simulink model "exp11_4"  (R2020a)
settings: Solver=FixedStepAuto  StartTime=0.0  StopTime=5  FixedStep=0.01  RelTol=1e-3
settings Model: Creator=Sing Ngai  LastModifiedBy=zengw

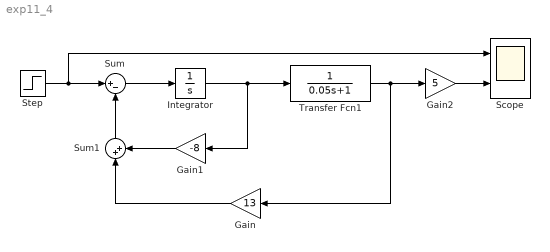
== system exp11_4 ==
  Gain : Gain  Gain=13
  Gain1 : Gain  Gain=-8
  Gain2 : Gain  Gain=5
  Integrator : Integrator
  Scope : Scope  NumInputPorts=2
  Step : Step  Before=1  SampleTime=0
  Sum : Sum  Inputs=|+-
  Sum1 : Sum  Inputs=|++
  Transfer Fcn1 : TransferFcn  Denominator=[0.05 1]
  wires:
  Step/1 -> Scope/1, Sum/1
  Sum/1 -> Integrator/1
  Integrator/1 -> Transfer Fcn1/1, Gain1/1
  Transfer Fcn1/1 -> Gain2/1, Gain/1
  Gain/1 -> Sum1/1
  Gain1/1 -> Sum1/2
  Sum1/1 -> Sum/2
  Gain2/1 -> Scope/2
